simulink model "Copter_Plane_h2g_V10g"  (R2020b)
settings: Solver=ode1  StartTime=0.0  StopTime=6  FixedStep=dt  MaxStep=Ts  RelTol=1e-3
values from neighbouring files (symbols this model uses):
  HD = 180/pi    (= 57.2957795131)    [mode_data.m]
  POSCONTROL_ACC_Z_D = 0.3    [data_devg2.m]
  POSCONTROL_ACC_Z_P = 0.9    [data_devg2.m]
  POSCONTROL_VEL_XY_D = 0.12    [data_devg2.m]
  POSCONTROL_VEL_XY_P = 1.1    [data_devg2.m]
undefined symbols (not defined in the file or in its folder): accel_target, attitude_target_euler_angle, center_WP, curr_pos, curr_vel, GRAVITY_MSS, gyro_x, gyro_y, gyro_z, J, k_aileron, k_aileronL, k_aileronR, k_elevator, k_flap, k_rudder, m_kg, Newton, pid_vel_xy_derivative, pid_vel_xy_input, pid_vel_xy_integrator, pitch, pos_target, pwm_out, pwm_tail, Raphson, rate_target_ang_vel, roll, tail_tilt, Vehicle, vel_desired, vel_target, yaw
libraries: sharedutil x11, sharedtransform x5, shared6dofsys x3, simulink x2, aerolibasang x1
(part 4 of 5)

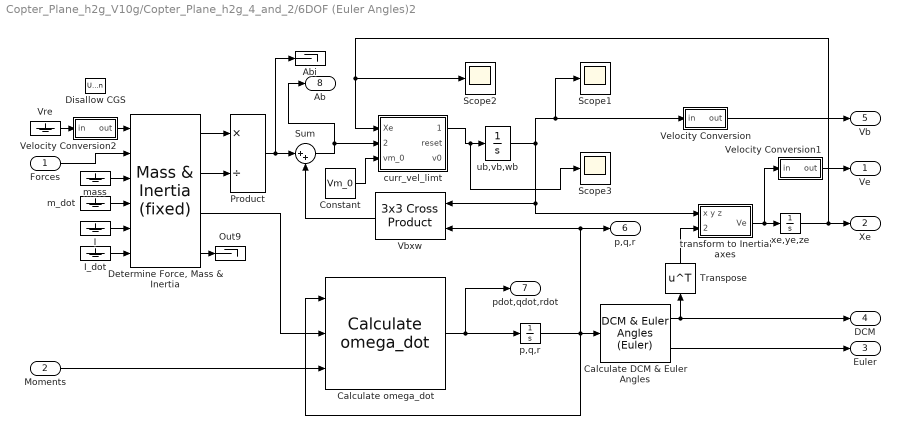
== system Copter_Plane_h2g_V10g/Copter_Plane_h2g_4_and_2/6DOF (Euler Angles)2 ==
  Forces : Inport  Unit=N  PortDimensions=3
  Moments : Inport  Port=2  Unit=N*m  PortDimensions=3
  Abi : Terminator
  Calculate DCM & Euler Angles : shared6dofsys/DCM & Euler Angles (Euler)  aMode=aMode
      settings: SourceProductBaseCode=AE,PW,MT,UV,VE,VP
  Calculate omega_dot : shared6dofsys/Calculate omega_dot  aMode=aMode
      settings: SourceProductBaseCode=AE,PW,MT,UV,VE,VP
  Constant : Constant  Value=Vm_0
  "Determine Force, Mass & Inertia" : shared6dofsys/Mass & Inertia (fixed)  aMode=aMode
      settings: SourceProductBaseCode=AE,PW,MT,UV,VE,VP
  Disallow CGS : UnitConfiguration  UnitSystemsStr=English,SI,SI (extended)  AllowAllUnitSystems=off
  I : Ground
  I_dot : Ground
  Out9 : Terminator
  Product : Product  Inputs=*/  SaturateOnIntegerOverflow=on  OutDataTypeStr=Inherit: Same as first input
  Scope1 : Scope
  Scope2 : Scope
  Scope3 : Scope
  Sum : Sum  Inputs=|++  SaturateOnIntegerOverflow=on
  Transpose : Math  Operator=transpose  SignedPower=on  SaturateOnIntegerOverflow=on
  Vbxw : sharedutil/3x3 Cross Product  aMode=aMode
      settings: SourceProductBaseCode=AE,PW,MT,UV,VE,VP
  Velocity Conversion : Subsystem
  Velocity Conversion1 : Subsystem
  Velocity Conversion2 : Subsystem
  Vre : Ground
  curr_vel_limt : MATLAB Function  TreatAsAtomicUnit=on
  m_dot : Ground
  mass : Ground
  "p,q,r " : Integrator  InitialCondition=pm_0  ContinuousStateAttributes=pm_statename
  "transform to Inertial axes " : Subsystem  mask(Vector Transformation){}
      mask Display: disp('L_EB')
  ub,vb,wb : Integrator  InitialCondition=Vm_0  UpperSaturationLimit=[inf inf 0]  ContinuousStateAttributes=Vm_statename
  xe,ye,ze : Integrator  InitialCondition=xme_0  ContinuousStateAttributes=xme_statename
  Ve : Outport  Unit=m/s  VectorParamsAs1DForOutWhenUnconnected=off
  Xe : Outport  Port=2  Unit=m  VectorParamsAs1DForOutWhenUnconnected=off
  Euler : Outport  Port=3  Unit=rad  VectorParamsAs1DForOutWhenUnconnected=off
  DCM : Outport  Port=4  Unit=1  VectorParamsAs1DForOutWhenUnconnected=off
  Vb : Outport  Port=5  Unit=m/s  VectorParamsAs1DForOutWhenUnconnected=off
  p,q,r : Outport  Port=6  Unit=rad/s  VectorParamsAs1DForOutWhenUnconnected=off
  pdot,qdot,rdot : Outport  Port=7  Unit=rad/s^2  VectorParamsAs1DForOutWhenUnconnected=off
  Ab : Outport  Port=8  Unit=m/s^2  VectorParamsAs1DForOutWhenUnconnected=off
  wires:
  Velocity Conversion1/1(out) -> Ve/1
  Sum/1 -> Ab/1, curr_vel_limt/2(accel_in)
  ub,vb,wb/1 -> "transform to Inertial axes "/1(x y z), Vbxw/1, Scope1/1, Velocity Conversion/1(in)
  Velocity Conversion/1(out) -> Vb/1
  Velocity Conversion2/1(out) -> "Determine Force, Mass & Inertia"/1
  Vre/1 -> Velocity Conversion2/1(in)
  "Determine Force, Mass & Inertia"/1 -> Product/1
  I_dot/1 -> "Determine Force, Mass & Inertia"/6
  I/1 -> "Determine Force, Mass & Inertia"/5
  Calculate omega_dot/1 -> "p,q,r "/1, pdot,qdot,rdot/1
  "Determine Force, Mass & Inertia"/4 -> Out9/1
  m_dot/1 -> "Determine Force, Mass & Inertia"/4
  "Determine Force, Mass & Inertia"/2 -> Product/2
  mass/1 -> "Determine Force, Mass & Inertia"/3
  Transpose/1 -> "transform to Inertial axes "/2(transform coefficients)
  Calculate DCM & Euler Angles/1 -> Transpose/1, DCM/1
  Product/1 -> Sum/1, Abi/1
  Forces/1 -> "Determine Force, Mass & Inertia"/2
  Moments/1 -> Calculate omega_dot/3
  "p,q,r "/1 -> Calculate DCM & Euler Angles/1, Calculate omega_dot/1, p,q,r/1, Vbxw/2
  "transform to Inertial axes "/1(Ve) -> xe,ye,ze/1, Velocity Conversion1/1(in)
  xe,ye,ze/1 -> Scope2/1, curr_vel_limt/1(Xe), Xe/1
  Vbxw/1 -> Sum/2
  Calculate DCM & Euler Angles/2 -> Euler/1
  "Determine Force, Mass & Inertia"/3 -> Calculate omega_dot/2
  curr_vel_limt/1(accel_o) -> Scope3/1, ub,vb,wb/1
  Constant/1 -> curr_vel_limt/3(vm_0)

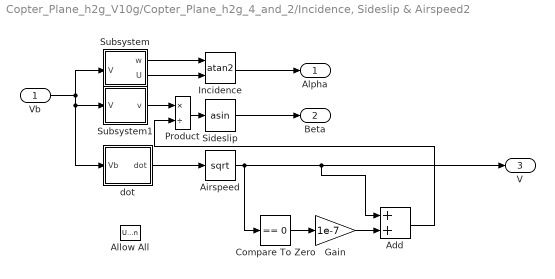
== system Copter_Plane_h2g_V10g/Copter_Plane_h2g_4_and_2/Incidence, Sideslip & Airspeed2 ==
  Vb : Inport
  Add : Sum
  Airspeed : Sqrt  AlgorithmType=Newton-Raphson  SaturateOnIntegerOverflow=on
  Allow All : UnitConfiguration  UnitSystemsStr=English,SI,SI (extended)  AllowAllUnitSystems=off
  Compare To Zero : simulink/Logic and Bit Operations/Compare To Zero  relop===  OutDataTypeStr=boolean
  Gain : Gain  Gain=1e-7
  Incidence : Trigonometry  Operator=atan2
  Product : Product  Inputs=*/  SaturateOnIntegerOverflow=on  OutDataTypeStr=Inherit: Same as first input
  Sideslip : Trigonometry  Operator=asin
  Subsystem : Subsystem
  Subsystem1 : Subsystem
  dot : Subsystem
  Alpha : Outport  Unit=rad  InitialOutput=0  VectorParamsAs1DForOutWhenUnconnected=off
  Beta : Outport  Port=2  Unit=rad  InitialOutput=0  VectorParamsAs1DForOutWhenUnconnected=off
  V : Outport  Port=3  InitialOutput=0  VectorParamsAs1DForOutWhenUnconnected=off
  wires:
  Product/1 -> Sideslip/1
  Subsystem/1(w) -> Incidence/1
  Subsystem/2(U) -> Incidence/2
  dot/1(dot) -> Airspeed/1
  Airspeed/1 -> Compare To Zero/1, Add/1, V/1
  Incidence/1 -> Alpha/1
  Vb/1 -> Subsystem/1(V), Subsystem1/1(V), dot/1(Vb)
  Sideslip/1 -> Beta/1
  Subsystem1/1(v) -> Product/1
  Compare To Zero/1 -> Gain/1
  Gain/1 -> Add/2
  Add/1 -> Product/2

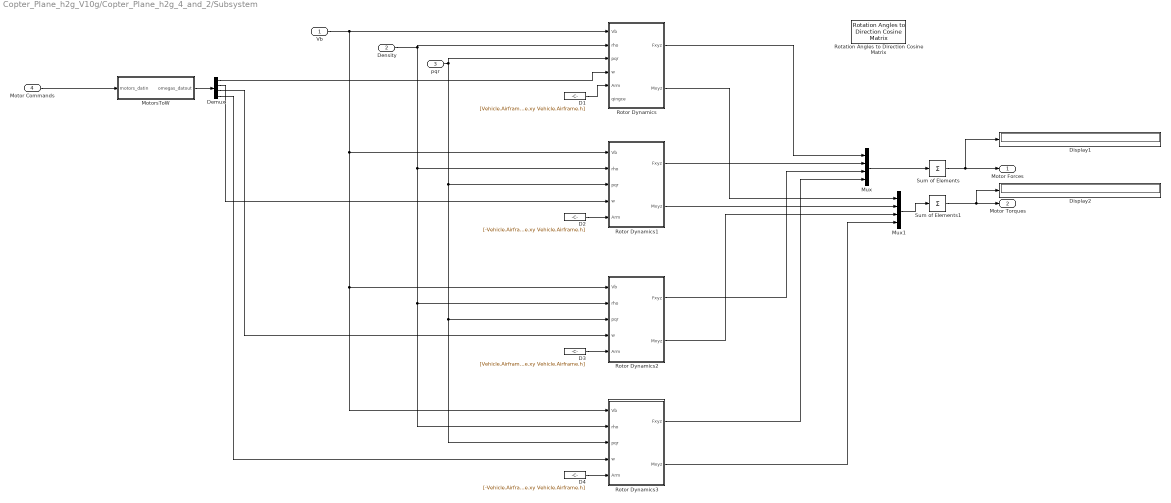
== system Copter_Plane_h2g_V10g/Copter_Plane_h2g_4_and_2/Subsystem ==
  Vb : Inport
  Density : Inport  Port=2
  pqr : Inport  Port=3
  Motor Commands : Inport  Port=4
  D1 : Constant  Value=[Vehicle.Airframe.xy +Vehicle.Airframe.xy Vehicle.Airframe.h]
  D2 : Constant  Value=[-Vehicle.Airframe.xy -Vehicle.Airframe.xy Vehicle.Airframe.h]
  D3 : Constant  Value=[Vehicle.Airframe.xy -Vehicle.Airframe.xy Vehicle.Airframe.h]
  D4 : Constant  Value=[-Vehicle.Airframe.xy Vehicle.Airframe.xy Vehicle.Airframe.h]
  Demux : Demux
  Display1 : Display
  Display2 : Display
  MotorsToW : Subsystem
  Mux : Mux
  Mux1 : Mux
  Rotation Angles to Direction Cosine Matrix : sharedtransform/Rotation Angles to Direction Cosine Matrix  rotationOrder=YZX  aMode=aMode
      settings: SourceProductBaseCode=AE,PW,MT,UV,VE,VP
  Rotor Dynamics : Subsystem  AncestorBlock=dynamicsLibrary/Rotor Dynamics  TreatAsAtomicUnit=on
      mask init:
      | aeroicon('aeroblk');
      settings: RTWFcnNameOpts=Use subsystem name  RTWFileNameOpts=Use function name
  Rotor Dynamics1 : Subsystem  AncestorBlock=dynamicsLibrary/Rotor Dynamics  TreatAsAtomicUnit=on
      mask init:
      | aeroicon('aeroblk');
      settings: RTWFcnNameOpts=Use subsystem name  RTWFileNameOpts=Use function name
  Rotor Dynamics2 : Subsystem  AncestorBlock=dynamicsLibrary/Rotor Dynamics  TreatAsAtomicUnit=on
      mask init:
      | aeroicon('aeroblk');
      settings: RTWFcnNameOpts=Use subsystem name  RTWFileNameOpts=Use function name
  Rotor Dynamics3 : Subsystem  AncestorBlock=dynamicsLibrary/Rotor Dynamics  TreatAsAtomicUnit=on
      mask init:
      | aeroicon('aeroblk');
      settings: RTWFcnNameOpts=Use subsystem name  RTWFileNameOpts=Use function name
  Sum of Elements : Sum  Inputs=+  CollapseMode=Specified dimension  CollapseDim=2
  Sum of Elements1 : Sum  Inputs=+  CollapseMode=Specified dimension  CollapseDim=2
  Motor Forces : Outport  Unit=N  VectorParamsAs1DForOutWhenUnconnected=off
  Motor Torques : Outport  Port=2  Unit=N*m  VectorParamsAs1DForOutWhenUnconnected=off
  wires:
  D4/1 -> Rotor Dynamics3/5(Arm)
  Sum of Elements1/1 -> Display2/1, Motor Torques/1
  D3/1 -> Rotor Dynamics2/5(Arm)
  Sum of Elements/1 -> Display1/1, Motor Forces/1
  D1/1 -> Rotor Dynamics/5(Arm)
  Mux1/1 -> Sum of Elements1/1
  Mux/1 -> Sum of Elements/1
  D2/1 -> Rotor Dynamics1/5(Arm)
  Motor Commands/1 -> MotorsToW/1(motors_datin)
  MotorsToW/1(omegas_datout) -> Demux/1
  Vb/1 -> Rotor Dynamics/1(Vb), Rotor Dynamics2/1(Vb), Rotor Dynamics3/1(Vb), Rotor Dynamics1/1(Vb)
  Density/1 -> Rotor Dynamics/2(rho), Rotor Dynamics2/2(rho), Rotor Dynamics3/2(rho), Rotor Dynamics1/2(rho)
  pqr/1 -> Rotor Dynamics/3(pqr), Rotor Dynamics2/3(pqr), Rotor Dynamics3/3(pqr), Rotor Dynamics1/3(pqr)
  Demux/1 -> Rotor Dynamics/4(w)
  Demux/2 -> Rotor Dynamics1/4(w)
  Demux/3 -> Rotor Dynamics2/4(w)
  Demux/4 -> Rotor Dynamics3/4(w)
  Rotor Dynamics/1(Fxyz) -> Mux/1
  Rotor Dynamics1/1(Fxyz) -> Mux/2
  Rotor Dynamics2/1(Fxyz) -> Mux/3
  Rotor Dynamics3/1(Fxyz) -> Mux/4
  Rotor Dynamics1/2(Mxyz) -> Mux1/2
  Rotor Dynamics2/2(Mxyz) -> Mux1/3
  Rotor Dynamics/2(Mxyz) -> Mux1/1
  Rotor Dynamics3/2(Mxyz) -> Mux1/4

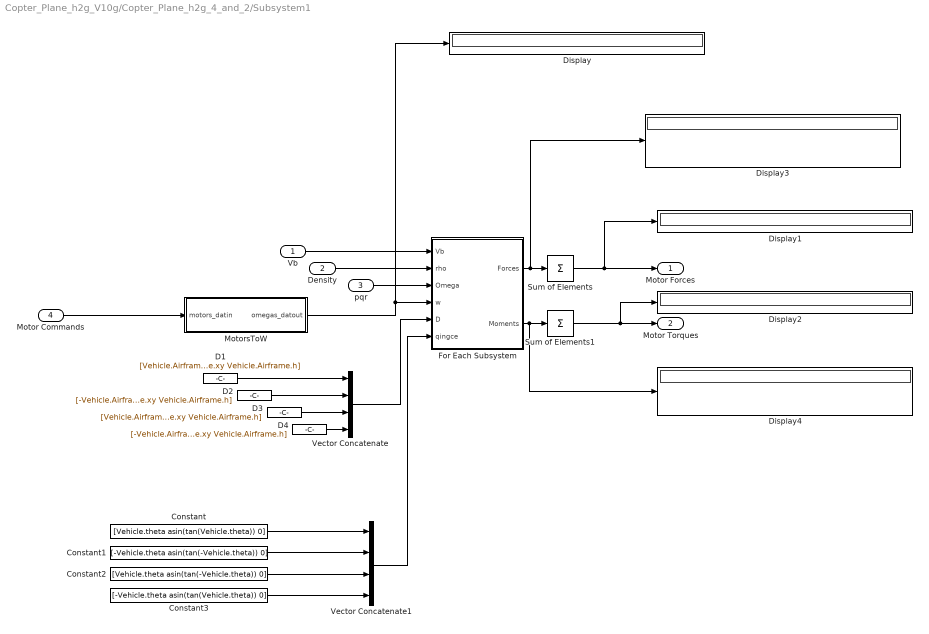
== system Copter_Plane_h2g_V10g/Copter_Plane_h2g_4_and_2/Subsystem1 ==
  Vb : Inport
  Density : Inport  Port=2
  pqr : Inport  Port=3
  Motor Commands : Inport  Port=4
  Constant : Constant  Value=[Vehicle.theta asin(tan(Vehicle.theta)) 0]
  Constant1 : Constant  Value=[-Vehicle.theta asin(tan(-Vehicle.theta)) 0]
  Constant2 : Constant  Value=[Vehicle.theta asin(tan(-Vehicle.theta)) 0]
  Constant3 : Constant  Value=[-Vehicle.theta asin(tan(Vehicle.theta)) 0]
  D1 : Constant  Value=[Vehicle.Airframe.xy +Vehicle.Airframe.xy Vehicle.Airframe.h]
  D2 : Constant  Value=[-Vehicle.Airframe.xy -Vehicle.Airframe.xy Vehicle.Airframe.h]
  D3 : Constant  Value=[Vehicle.Airframe.xy -Vehicle.Airframe.xy Vehicle.Airframe.h]
  D4 : Constant  Value=[-Vehicle.Airframe.xy Vehicle.Airframe.xy Vehicle.Airframe.h]
  Display{,1..4} (5 alike) : Display
  For Each Subsystem : Subsystem  TreatAsAtomicUnit=on
  MotorsToW : Subsystem
  Sum of Elements : Sum  Inputs=+  CollapseMode=Specified dimension  CollapseDim=2
  Sum of Elements1 : Sum  Inputs=+  CollapseMode=Specified dimension  CollapseDim=2
  Vector Concatenate : Concatenate  NumInputs=4  Mode=Multidimensional array  ConcatenateDimension=2
  Vector Concatenate1 : Concatenate  NumInputs=4  Mode=Multidimensional array  ConcatenateDimension=2
  Motor Forces : Outport  Unit=N  VectorParamsAs1DForOutWhenUnconnected=off
  Motor Torques : Outport  Port=2  Unit=N*m  VectorParamsAs1DForOutWhenUnconnected=off
  wires:
  Vector Concatenate/1 -> For Each Subsystem/5(D)
  Density/1 -> For Each Subsystem/2(rho)
  D4/1 -> Vector Concatenate/4
  Vb/1 -> For Each Subsystem/1(Vb)
  Sum of Elements1/1 -> Display2/1, Motor Torques/1
  D3/1 -> Vector Concatenate/3
  Sum of Elements/1 -> Display1/1, Motor Forces/1
  pqr/1 -> For Each Subsystem/3(Omega)
  D1/1 -> Vector Concatenate/1
  For Each Subsystem/2(Moments) -> Display4/1, Sum of Elements1/1
  For Each Subsystem/1(Forces) -> Display3/1, Sum of Elements/1
  D2/1 -> Vector Concatenate/2
  MotorsToW/1(omegas_datout) -> Display/1, For Each Subsystem/4(w)
  Motor Commands/1 -> MotorsToW/1(motors_datin)
  Vector Concatenate1/1 -> For Each Subsystem/6(qingce)
  Constant/1 -> Vector Concatenate1/1
  Constant1/1 -> Vector Concatenate1/2
  Constant2/1 -> Vector Concatenate1/3
  Constant3/1 -> Vector Concatenate1/4

== system Copter_Plane_h2g_V10g/Copter_Plane_h2g_4_and_2/6DOF (Euler Angles)2/Velocity Conversion ==
  in : Inport  Unit=m/s
  Unit Conversion : UnitConversion
  out : Outport  VectorParamsAs1DForOutWhenUnconnected=off
  wires:
  Unit Conversion/1 -> out/1
  in/1 -> Unit Conversion/1

== system Copter_Plane_h2g_V10g/Copter_Plane_h2g_4_and_2/6DOF (Euler Angles)2/Velocity Conversion1 ==
  in : Inport  Unit=m/s
  Unit Conversion : UnitConversion
  out : Outport  VectorParamsAs1DForOutWhenUnconnected=off
  wires:
  Unit Conversion/1 -> out/1
  in/1 -> Unit Conversion/1

== system Copter_Plane_h2g_V10g/Copter_Plane_h2g_4_and_2/6DOF (Euler Angles)2/Velocity Conversion2 ==
  in : Inport  Unit=m/s
  Unit Conversion : UnitConversion
  out : Outport  Unit=m/s  VectorParamsAs1DForOutWhenUnconnected=off
  wires:
  Unit Conversion/1 -> out/1
  in/1 -> Unit Conversion/1

== system Copter_Plane_h2g_V10g/Copter_Plane_h2g_4_and_2/6DOF (Euler Angles)2/transform to Inertial axes  ==
  x y z : Inport
  transform coefficients : Inport  Port=2
  Product : Product  Multiplication=Matrix(*)  InputSameDT=on  SaturateOnIntegerOverflow=on  OutDataTypeStr=Inherit: Same as first input
  Reshape1 : Reshape  OutputDimensionality=Column vector (2-D)
  Reshape2 : Reshape
  Ve : Outport  VectorParamsAs1DForOutWhenUnconnected=off
  wires:
  Reshape2/1 -> Ve/1
  Reshape1/1 -> Product/2
  x y z/1 -> Reshape1/1
  transform coefficients/1 -> Product/1
  Product/1 -> Reshape2/1

== system Copter_Plane_h2g_V10g/Copter_Plane_h2g_4_and_2/Incidence, Sideslip & Airspeed2/Subsystem ==
  V : Inport
  Demux1 : Demux  Outputs=3
      settings: DisplayOption=none
  Terminator : Terminator
  w : Outport  VectorParamsAs1DForOutWhenUnconnected=off
  U : Outport  Port=2  VectorParamsAs1DForOutWhenUnconnected=off
  wires:
  Demux1/3 -> w/1
  Demux1/2 -> Terminator/1
  V/1 -> Demux1/1
  Demux1/1 -> U/1

== system Copter_Plane_h2g_V10g/Copter_Plane_h2g_4_and_2/Incidence, Sideslip & Airspeed2/Subsystem1 ==
  V : Inport
  Demux1 : Demux  Outputs=3
      settings: DisplayOption=none
  Terminator : Terminator
  Terminator1 : Terminator
  v : Outport  VectorParamsAs1DForOutWhenUnconnected=off
  wires:
  Demux1/1 -> Terminator/1
  Demux1/3 -> Terminator1/1
  V/1 -> Demux1/1
  Demux1/2 -> v/1

== system Copter_Plane_h2g_V10g/Copter_Plane_h2g_4_and_2/Incidence, Sideslip & Airspeed2/dot ==
  Vb : Inport
  Demux1 : Demux  Outputs=3
  Product : Product  RndMeth=Zero
  Product1 : Product  RndMeth=Zero
  Product2 : Product  RndMeth=Zero
  Sum : Sum  Inputs=+++
  dot : Outport  VectorParamsAs1DForOutWhenUnconnected=off
  wires:
  Product2/1 -> Sum/3
  Demux1/3 -> Product2/2, Product2/1
  Product/1 -> Sum/1
  Product1/1 -> Sum/2
  Sum/1 -> dot/1
  Vb/1 -> Demux1/1
  Demux1/1 -> Product/2, Product/1
  Demux1/2 -> Product1/1, Product1/2

== system Copter_Plane_h2g_V10g/Copter_Plane_h2g_4_and_2/Subsystem/MotorsToW ==
  motors_datin : Inport
  Motordirections1 : Gain  Gain=[1 1 -1 -1]  ParamDataTypeStr=single  OutDataTypeStr=Inherit: Inherit via back propagation  SaturateOnIntegerOverflow=on
  Saturation5 : Saturate  UpperLimit=1  LowerLimit=realmin  OutDataTypeStr=Inherit: Inherit via back propagation
  motorsToW2_Gain : Gain  Gain=Vehicle.Motor.commandToWGain  ParamDataTypeStr=single  OutDataTypeStr=Inherit: Inherit via back propagation  SaturateOnIntegerOverflow=on
  motorsToW2_Gain1 : Gain  Gain=2*pi/60  ParamDataTypeStr=single  OutDataTypeStr=Inherit: Inherit via back propagation  SaturateOnIntegerOverflow=on
  omegas_datout : Outport  VectorParamsAs1DForOutWhenUnconnected=off
  wires:
  Saturation5/1 -> Motordirections1/1
  Motordirections1/1 -> motorsToW2_Gain/1
  motors_datin/1 -> Saturation5/1
  motorsToW2_Gain/1 -> motorsToW2_Gain1/1
  motorsToW2_Gain1/1 -> omegas_datout/1

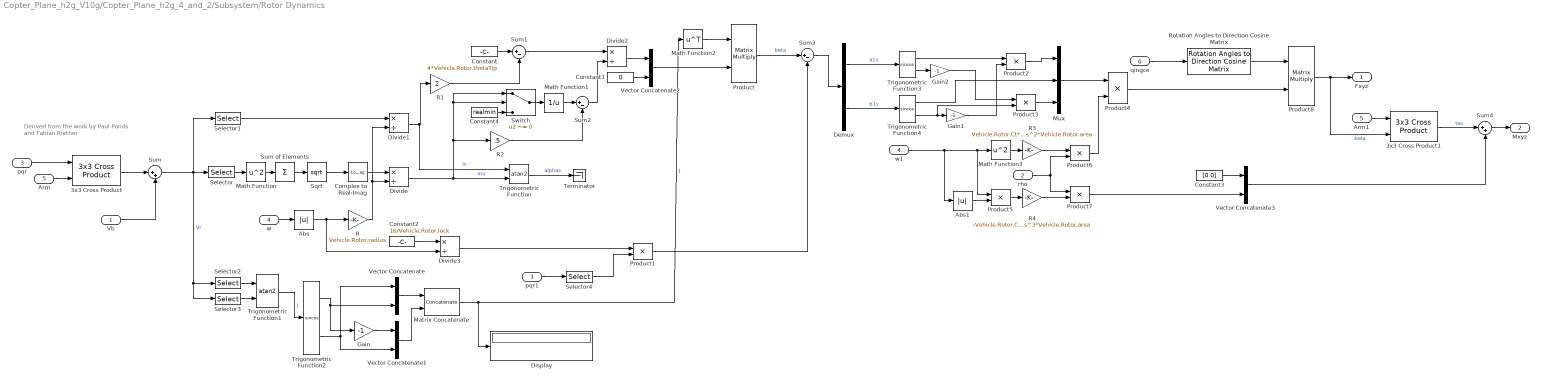
== system Copter_Plane_h2g_V10g/Copter_Plane_h2g_4_and_2/Subsystem/Rotor Dynamics ==
  note: Derived from the work by Paul Ponds
      | and Fabian Riether
  Vb : Inport  PortDimensions=3
  rho : Inport  Port=2  PortDimensions=1
  pqr : Inport  Port=3  PortDimensions=3
  w : Inport  Port=4  PortDimensions=[1 1]
  Arm : Inport  Port=5  PortDimensions=[3 1]
  qingce : Inport  Port=6  PortDimensions=[3 1]
  3x3 Cross Product : sharedutil/3x3 Cross Product  aMode=aMode
      settings: SourceProductBaseCode=AE,PW,MT,UV,VE,VP
  3x3 Cross Product1 : sharedutil/3x3 Cross Product  aMode=aMode
      settings: SourceProductBaseCode=AE,PW,MT,UV,VE,VP
  Abs : Abs
  Abs1 : Abs
  Arm1 : InportShadow  Port=5  PortDimensions=[3 1]
  Complex to Real-Imag : ComplexToRealImag  Output=Real
  Constant : Constant  Value=4*Vehicle.Rotor.thetaTip
  Constant1 : Constant  Value=0
  Constant2 : Constant  Value=16/Vehicle.Rotor.lock
  Constant3 : Constant  Value=[0 0]
  Constant4 : Constant  Value=realmin
  Demux : Demux  Outputs=2
  Display : Display
  Divide{,1..3} (4 alike) : Product  Inputs=*/
  Gain : Gain  Gain=-1
  Gain1 : Gain  Gain=-1
  Gain2 : Gain  Gain=-1
  Math Function : Math  Operator=square  SignedPower=on  SaturateOnIntegerOverflow=on
  Math Function1 : Math  Operator=reciprocal  SignedPower=on  SaturateOnIntegerOverflow=on
  Math Function2 : Math  Operator=transpose  SignedPower=on  SaturateOnIntegerOverflow=on
  Math Function3 : Math  Operator=square  SignedPower=on  SaturateOnIntegerOverflow=on
  Matrix Concatenate : Concatenate  Mode=Multidimensional array  ConcatenateDimension=2
  Mux : Mux  Inputs=3
  Product : Product  Multiplication=Matrix(*)
  Product{1..7} (7 alike) : Product
  Product8 : Product  Multiplication=Matrix(*)
  R : Gain  Gain=Vehicle.Rotor.radius
  R1 : Gain  Gain=2
  R2 : Gain  Gain=.5
  R3 : Gain  Gain=Vehicle.Rotor.Ct*Vehicle.Rotor.radius^2*Vehicle.Rotor.area
  R4 : Gain  Gain=-Vehicle.Rotor.Cq*Vehicle.Rotor.radius^3*Vehicle.Rotor.area
  Rotation Angles to Direction Cosine Matrix : sharedtransform/Rotation Angles to Direction Cosine Matrix  rotationOrder=YXZ  aMode=aMode
      settings: SourceProductBaseCode=AE,PW,MT,UV,VE,VP
  Selector : Selector  InputPortWidth=3  IndexOptions=Index vector (dialog)  Indices=[1 2]  OutputSizes=1
  Selector1 : Selector  InputPortWidth=3  IndexOptions=Index vector (dialog)  Indices=[3]  OutputSizes=1
  Selector2 : Selector  InputPortWidth=3  IndexOptions=Index vector (dialog)  Indices=[2]  OutputSizes=1
  Selector3 : Selector  InputPortWidth=3  IndexOptions=Index vector (dialog)  Indices=[1]  OutputSizes=1
  Selector4 : Selector  InputPortWidth=3  IndexOptions=Index vector (dialog)  Indices=[2 1]  OutputSizes=1
  Sqrt : Sqrt  OutputSignalType=complex  SaturateOnIntegerOverflow=on
  Sum : Sum  Inputs=|++
  Sum of Elements : Sum  Inputs=+
  Sum1 : Sum  Inputs=|+-
  Sum2 : Sum  Inputs=|+-
  Sum3 : Sum  Inputs=|+-
  Sum4 : Sum  Inputs=|++
  Switch : Switch  Criteria=u2 ~= 0
  Terminator : Terminator
  Trigonometric Function : Trigonometry  Operator=atan2
  Trigonometric Function1 : Trigonometry  Operator=atan2
  Trigonometric Function2 : Trigonometry  Operator=sincos
  Trigonometric Function3 : Trigonometry  Operator=sincos
  Trigonometric Function4 : Trigonometry  Operator=sincos
  Vector Concatenate{,1..3} (4 alike) : Concatenate
  pqr1 : InportShadow  Port=3  PortDimensions=3
  w1 : InportShadow  Port=4  PortDimensions=[1 1]
  Fxyz : Outport  PortDimensions=[3 1]  VectorParamsAs1DForOutWhenUnconnected=off
  Mxyz : Outport  Port=2  PortDimensions=[3 1]  VectorParamsAs1DForOutWhenUnconnected=off
  wires:
  Complex to Real-Imag/1 -> Divide/1
  Sqrt/1 -> Complex to Real-Imag/1
  Constant4/1 -> Switch/3
  Switch/1 -> Math Function1/1
  Product1/1 -> Sum3/2
  rho/1 -> Product7/1, Product6/2
  Product7/1 -> Vector Concatenate3/2
  Product6/1 -> Product4/2
  Sum4/1 -> Mxyz/1
  3x3 Cross Product1/1 -> Sum4/1  "tau"
  Product4/1 -> Product8/2
  Arm1/1 -> 3x3 Cross Product1/1
  Vector Concatenate3/1 -> Sum4/2
  Constant3/1 -> Vector Concatenate3/1
  R4/1 -> Product7/2
  Product5/1 -> R4/1
  Abs1/1 -> Product5/2
  R3/1 -> Product6/1
  Mux/1 -> Product4/1
  Gain2/1 -> Product3/1
  Product3/1 -> Mux/3
  Trigonometric Function3/2 -> Gain2/1
  Trigonometric Function4/1 -> Mux/2
  Product2/1 -> Mux/1
  Trigonometric Function3/1 -> Product2/1
  Gain1/1 -> Product2/2
  Trigonometric Function4/2 -> Gain1/1, Product3/2
  Demux/2 -> Trigonometric Function4/1  "b1s"
  Demux/1 -> Trigonometric Function3/1  "a1s"
  Sum3/1 -> Demux/1
  Math Function3/1 -> R3/1
  w1/1 -> Math Function3/1, Product5/1, Abs1/1
  Divide3/1 -> Product1/1
  Abs/1 -> R/1, Divide3/2
  Selector4/1 -> Product1/2
  pqr1/1 -> Selector4/1
  Constant2/1 -> Divide3/1
  Product/1 -> Sum3/1  "beta"
  Math Function2/1 -> Product/1
  Vector Concatenate2/1 -> Product/2
  Constant1/1 -> Vector Concatenate2/2
  Divide2/1 -> Vector Concatenate2/1
  Sum2/1 -> Divide2/2
  R2/1 -> Sum2/2
  Math Function1/1 -> Sum2/1
  Sum1/1 -> Divide2/1
  R1/1 -> Sum1/2
  Constant/1 -> Sum1/1
  Matrix Concatenate/1 -> Display/1, Math Function2/1  "J"
  Vector Concatenate1/1 -> Matrix Concatenate/2
  Vector Concatenate/1 -> Matrix Concatenate/1
  Trigonometric Function2/1 -> Gain/1, Vector Concatenate/2
  Gain/1 -> Vector Concatenate1/1
  Trigonometric Function2/2 -> Vector Concatenate/1, Vector Concatenate1/2
  Trigonometric Function1/1 -> Trigonometric Function2/1  "j"
  Selector3/1 -> Trigonometric Function1/2
  Selector2/1 -> Trigonometric Function1/1
  Trigonometric Function/1 -> Terminator/1  "alphas"
  Divide1/1 -> Trigonometric Function/1, R1/1  "lc"
  Selector1/1 -> Divide1/1
  Divide/1 -> Trigonometric Function/2, Switch/1, Switch/2, R2/1  "mu"
  R/1 -> Divide/2, Divide1/2
  w/1 -> Abs/1
  Arm/1 -> 3x3 Cross Product/2
  pqr/1 -> 3x3 Cross Product/1
  Sum of Elements/1 -> Sqrt/1
  Math Function/1 -> Sum of Elements/1
  Selector/1 -> Math Function/1
  Sum/1 -> Selector/1, Selector1/1, Selector2/1, Selector3/1  "Vr"
  Vb/1 -> Sum/2
  3x3 Cross Product/1 -> Sum/1
  Rotation Angles to Direction Cosine Matrix/1 -> Product8/1
  Product8/1 -> 3x3 Cross Product1/2, Fxyz/1  "beta"
  qingce/1 -> Rotation Angles to Direction Cosine Matrix/1

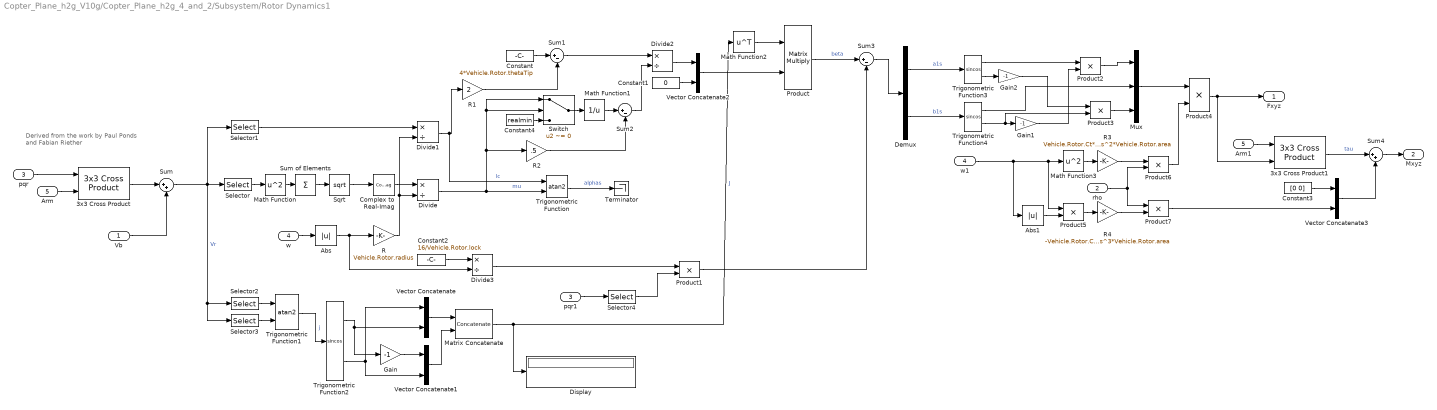
== system Copter_Plane_h2g_V10g/Copter_Plane_h2g_4_and_2/Subsystem/Rotor Dynamics1 ==
  note: Derived from the work by Paul Ponds
      | and Fabian Riether
  Vb : Inport  PortDimensions=3
  rho : Inport  Port=2  PortDimensions=1
  pqr : Inport  Port=3  PortDimensions=3
  w : Inport  Port=4  PortDimensions=[1 1]
  Arm : Inport  Port=5  PortDimensions=[3 1]
  3x3 Cross Product : sharedutil/3x3 Cross Product  aMode=aMode
      settings: SourceProductBaseCode=AE,PW,MT,UV,VE,VP
  3x3 Cross Product1 : sharedutil/3x3 Cross Product  aMode=aMode
      settings: SourceProductBaseCode=AE,PW,MT,UV,VE,VP
  Abs : Abs
  Abs1 : Abs
  Arm1 : InportShadow  Port=5  PortDimensions=[3 1]
  Complex to Real-Imag : ComplexToRealImag  Output=Real
  Constant : Constant  Value=4*Vehicle.Rotor.thetaTip
  Constant1 : Constant  Value=0
  Constant2 : Constant  Value=16/Vehicle.Rotor.lock
  Constant3 : Constant  Value=[0 0]
  Constant4 : Constant  Value=realmin
  Demux : Demux  Outputs=2
  Display : Display
  Divide{,1..3} (4 alike) : Product  Inputs=*/
  Gain : Gain  Gain=-1
  Gain1 : Gain  Gain=-1
  Gain2 : Gain  Gain=-1
  Math Function : Math  Operator=square  SignedPower=on  SaturateOnIntegerOverflow=on
  Math Function1 : Math  Operator=reciprocal  SignedPower=on  SaturateOnIntegerOverflow=on
  Math Function2 : Math  Operator=transpose  SignedPower=on  SaturateOnIntegerOverflow=on
  Math Function3 : Math  Operator=square  SignedPower=on  SaturateOnIntegerOverflow=on
  Matrix Concatenate : Concatenate  Mode=Multidimensional array  ConcatenateDimension=2
  Mux : Mux  Inputs=3
  Product : Product  Multiplication=Matrix(*)
  Product{1..7} (7 alike) : Product
  R : Gain  Gain=Vehicle.Rotor.radius
  R1 : Gain  Gain=2
  R2 : Gain  Gain=.5
  R3 : Gain  Gain=Vehicle.Rotor.Ct*Vehicle.Rotor.radius^2*Vehicle.Rotor.area
  R4 : Gain  Gain=-Vehicle.Rotor.Cq*Vehicle.Rotor.radius^3*Vehicle.Rotor.area
  Selector : Selector  InputPortWidth=3  IndexOptions=Index vector (dialog)  Indices=[1 2]  OutputSizes=1
  Selector1 : Selector  InputPortWidth=3  IndexOptions=Index vector (dialog)  Indices=[3]  OutputSizes=1
  Selector2 : Selector  InputPortWidth=3  IndexOptions=Index vector (dialog)  Indices=[2]  OutputSizes=1
  Selector3 : Selector  InputPortWidth=3  IndexOptions=Index vector (dialog)  Indices=[1]  OutputSizes=1
  Selector4 : Selector  InputPortWidth=3  IndexOptions=Index vector (dialog)  Indices=[2 1]  OutputSizes=1
  Sqrt : Sqrt  OutputSignalType=complex  SaturateOnIntegerOverflow=on
  Sum : Sum  Inputs=|++
  Sum of Elements : Sum  Inputs=+
  Sum1 : Sum  Inputs=|+-
  Sum2 : Sum  Inputs=|+-
  Sum3 : Sum  Inputs=|+-
  Sum4 : Sum  Inputs=|++
  Switch : Switch  Criteria=u2 ~= 0
  Terminator : Terminator
  Trigonometric Function : Trigonometry  Operator=atan2
  Trigonometric Function1 : Trigonometry  Operator=atan2
  Trigonometric Function2 : Trigonometry  Operator=sincos
  Trigonometric Function3 : Trigonometry  Operator=sincos
  Trigonometric Function4 : Trigonometry  Operator=sincos
  Vector Concatenate{,1..3} (4 alike) : Concatenate
  pqr1 : InportShadow  Port=3  PortDimensions=3
  w1 : InportShadow  Port=4  PortDimensions=[1 1]
  Fxyz : Outport  PortDimensions=[3 1]  VectorParamsAs1DForOutWhenUnconnected=off
  Mxyz : Outport  Port=2  PortDimensions=[3 1]  VectorParamsAs1DForOutWhenUnconnected=off
  wires:
  3x3 Cross Product/1 -> Sum/1
  Vb/1 -> Sum/2
  Sum/1 -> Selector3/1, Selector2/1, Selector1/1, Selector/1  "Vr"
  Selector/1 -> Math Function/1
  Math Function/1 -> Sum of Elements/1
  Sum of Elements/1 -> Sqrt/1
  pqr/1 -> 3x3 Cross Product/1
  Arm/1 -> 3x3 Cross Product/2
  w/1 -> Abs/1
  R/1 -> Divide1/2, Divide/2
  Divide/1 -> R2/1, Switch/2, Switch/1, Trigonometric Function/2  "mu"
  Selector1/1 -> Divide1/1
  Divide1/1 -> R1/1, Trigonometric Function/1  "lc"
  Trigonometric Function/1 -> Terminator/1  "alphas"
  Selector2/1 -> Trigonometric Function1/1
  Selector3/1 -> Trigonometric Function1/2
  Trigonometric Function1/1 -> Trigonometric Function2/1  "j"
  Trigonometric Function2/2 -> Vector Concatenate1/2, Vector Concatenate/1
  Gain/1 -> Vector Concatenate1/1
  Trigonometric Function2/1 -> Vector Concatenate/2, Gain/1
  Vector Concatenate/1 -> Matrix Concatenate/1
  Vector Concatenate1/1 -> Matrix Concatenate/2
  Matrix Concatenate/1 -> Math Function2/1, Display/1  "J"
  Constant/1 -> Sum1/1
  R1/1 -> Sum1/2
  Sum1/1 -> Divide2/1
  Math Function1/1 -> Sum2/1
  R2/1 -> Sum2/2
  Sum2/1 -> Divide2/2
  Divide2/1 -> Vector Concatenate2/1
  Constant1/1 -> Vector Concatenate2/2
  Vector Concatenate2/1 -> Product/2
  Math Function2/1 -> Product/1
  Product/1 -> Sum3/1  "beta"
  Constant2/1 -> Divide3/1
  pqr1/1 -> Selector4/1
  Selector4/1 -> Product1/2
  Abs/1 -> Divide3/2, R/1
  Divide3/1 -> Product1/1
  w1/1 -> Abs1/1, Product5/1, Math Function3/1
  Math Function3/1 -> R3/1
  Sum3/1 -> Demux/1
  Demux/1 -> Trigonometric Function3/1  "a1s"
  Demux/2 -> Trigonometric Function4/1  "b1s"
  Trigonometric Function4/2 -> Product3/2, Gain1/1
  Gain1/1 -> Product2/2
  Trigonometric Function3/1 -> Product2/1
  Product2/1 -> Mux/1
  Trigonometric Function4/1 -> Mux/2
  Trigonometric Function3/2 -> Gain2/1
  Product3/1 -> Mux/3
  Gain2/1 -> Product3/1
  Mux/1 -> Product4/1
  R3/1 -> Product6/1
  Abs1/1 -> Product5/2
  Product5/1 -> R4/1
  R4/1 -> Product7/2
  Constant3/1 -> Vector Concatenate3/1
  Vector Concatenate3/1 -> Sum4/2
  Arm1/1 -> 3x3 Cross Product1/1
  Product4/1 -> 3x3 Cross Product1/2, Fxyz/1
  3x3 Cross Product1/1 -> Sum4/1  "tau"
  Sum4/1 -> Mxyz/1
  Product6/1 -> Product4/2
  Product7/1 -> Vector Concatenate3/2
  rho/1 -> Product6/2, Product7/1
  Product1/1 -> Sum3/2
  Switch/1 -> Math Function1/1
  Constant4/1 -> Switch/3
  Sqrt/1 -> Complex to Real-Imag/1
  Complex to Real-Imag/1 -> Divide/1

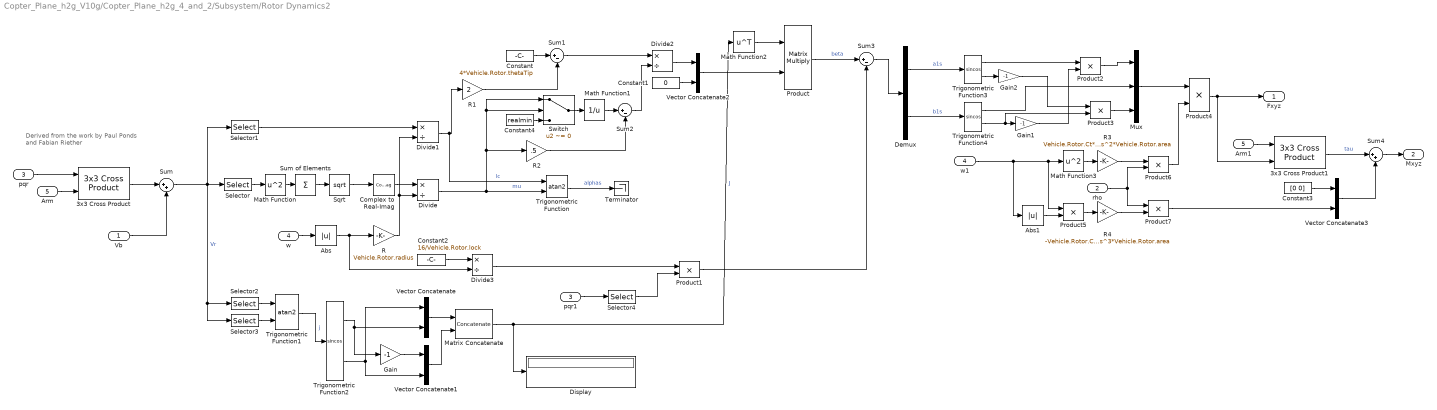
== system Copter_Plane_h2g_V10g/Copter_Plane_h2g_4_and_2/Subsystem/Rotor Dynamics2 ==
  note: Derived from the work by Paul Ponds
      | and Fabian Riether
  Vb : Inport  PortDimensions=3
  rho : Inport  Port=2  PortDimensions=1
  pqr : Inport  Port=3  PortDimensions=3
  w : Inport  Port=4  PortDimensions=[1 1]
  Arm : Inport  Port=5  PortDimensions=[3 1]
  3x3 Cross Product : sharedutil/3x3 Cross Product  aMode=aMode
      settings: SourceProductBaseCode=AE,PW,MT,UV,VE,VP
  3x3 Cross Product1 : sharedutil/3x3 Cross Product  aMode=aMode
      settings: SourceProductBaseCode=AE,PW,MT,UV,VE,VP
  Abs : Abs
  Abs1 : Abs
  Arm1 : InportShadow  Port=5  PortDimensions=[3 1]
  Complex to Real-Imag : ComplexToRealImag  Output=Real
  Constant : Constant  Value=4*Vehicle.Rotor.thetaTip
  Constant1 : Constant  Value=0
  Constant2 : Constant  Value=16/Vehicle.Rotor.lock
  Constant3 : Constant  Value=[0 0]
  Constant4 : Constant  Value=realmin
  Demux : Demux  Outputs=2
  Display : Display
  Divide{,1..3} (4 alike) : Product  Inputs=*/
  Gain : Gain  Gain=-1
  Gain1 : Gain  Gain=-1
  Gain2 : Gain  Gain=-1
  Math Function : Math  Operator=square  SignedPower=on  SaturateOnIntegerOverflow=on
  Math Function1 : Math  Operator=reciprocal  SignedPower=on  SaturateOnIntegerOverflow=on
  Math Function2 : Math  Operator=transpose  SignedPower=on  SaturateOnIntegerOverflow=on
  Math Function3 : Math  Operator=square  SignedPower=on  SaturateOnIntegerOverflow=on
  Matrix Concatenate : Concatenate  Mode=Multidimensional array  ConcatenateDimension=2
  Mux : Mux  Inputs=3
  Product : Product  Multiplication=Matrix(*)
  Product{1..7} (7 alike) : Product
  R : Gain  Gain=Vehicle.Rotor.radius
  R1 : Gain  Gain=2
  R2 : Gain  Gain=.5
  R3 : Gain  Gain=Vehicle.Rotor.Ct*Vehicle.Rotor.radius^2*Vehicle.Rotor.area
  R4 : Gain  Gain=-Vehicle.Rotor.Cq*Vehicle.Rotor.radius^3*Vehicle.Rotor.area
  Selector : Selector  InputPortWidth=3  IndexOptions=Index vector (dialog)  Indices=[1 2]  OutputSizes=1
  Selector1 : Selector  InputPortWidth=3  IndexOptions=Index vector (dialog)  Indices=[3]  OutputSizes=1
  Selector2 : Selector  InputPortWidth=3  IndexOptions=Index vector (dialog)  Indices=[2]  OutputSizes=1
  Selector3 : Selector  InputPortWidth=3  IndexOptions=Index vector (dialog)  Indices=[1]  OutputSizes=1
  Selector4 : Selector  InputPortWidth=3  IndexOptions=Index vector (dialog)  Indices=[2 1]  OutputSizes=1
  Sqrt : Sqrt  OutputSignalType=complex  SaturateOnIntegerOverflow=on
  Sum : Sum  Inputs=|++
  Sum of Elements : Sum  Inputs=+
  Sum1 : Sum  Inputs=|+-
  Sum2 : Sum  Inputs=|+-
  Sum3 : Sum  Inputs=|+-
  Sum4 : Sum  Inputs=|++
  Switch : Switch  Criteria=u2 ~= 0
  Terminator : Terminator
  Trigonometric Function : Trigonometry  Operator=atan2
  Trigonometric Function1 : Trigonometry  Operator=atan2
  Trigonometric Function2 : Trigonometry  Operator=sincos
  Trigonometric Function3 : Trigonometry  Operator=sincos
  Trigonometric Function4 : Trigonometry  Operator=sincos
  Vector Concatenate{,1..3} (4 alike) : Concatenate
  pqr1 : InportShadow  Port=3  PortDimensions=3
  w1 : InportShadow  Port=4  PortDimensions=[1 1]
  Fxyz : Outport  PortDimensions=[3 1]  VectorParamsAs1DForOutWhenUnconnected=off
  Mxyz : Outport  Port=2  PortDimensions=[3 1]  VectorParamsAs1DForOutWhenUnconnected=off
  wires:
  Complex to Real-Imag/1 -> Divide/1
  Sqrt/1 -> Complex to Real-Imag/1
  Constant4/1 -> Switch/3
  Switch/1 -> Math Function1/1
  Product1/1 -> Sum3/2
  rho/1 -> Product7/1, Product6/2
  Product7/1 -> Vector Concatenate3/2
  Product6/1 -> Product4/2
  Sum4/1 -> Mxyz/1
  3x3 Cross Product1/1 -> Sum4/1  "tau"
  Product4/1 -> Fxyz/1, 3x3 Cross Product1/2
  Arm1/1 -> 3x3 Cross Product1/1
  Vector Concatenate3/1 -> Sum4/2
  Constant3/1 -> Vector Concatenate3/1
  R4/1 -> Product7/2
  Product5/1 -> R4/1
  Abs1/1 -> Product5/2
  R3/1 -> Product6/1
  Mux/1 -> Product4/1
  Gain2/1 -> Product3/1
  Product3/1 -> Mux/3
  Trigonometric Function3/2 -> Gain2/1
  Trigonometric Function4/1 -> Mux/2
  Product2/1 -> Mux/1
  Trigonometric Function3/1 -> Product2/1
  Gain1/1 -> Product2/2
  Trigonometric Function4/2 -> Gain1/1, Product3/2
  Demux/2 -> Trigonometric Function4/1  "b1s"
  Demux/1 -> Trigonometric Function3/1  "a1s"
  Sum3/1 -> Demux/1
  Math Function3/1 -> R3/1
  w1/1 -> Math Function3/1, Product5/1, Abs1/1
  Divide3/1 -> Product1/1
  Abs/1 -> R/1, Divide3/2
  Selector4/1 -> Product1/2
  pqr1/1 -> Selector4/1
  Constant2/1 -> Divide3/1
  Product/1 -> Sum3/1  "beta"
  Math Function2/1 -> Product/1
  Vector Concatenate2/1 -> Product/2
  Constant1/1 -> Vector Concatenate2/2
  Divide2/1 -> Vector Concatenate2/1
  Sum2/1 -> Divide2/2
  R2/1 -> Sum2/2
  Math Function1/1 -> Sum2/1
  Sum1/1 -> Divide2/1
  R1/1 -> Sum1/2
  Constant/1 -> Sum1/1
  Matrix Concatenate/1 -> Display/1, Math Function2/1  "J"
  Vector Concatenate1/1 -> Matrix Concatenate/2
  Vector Concatenate/1 -> Matrix Concatenate/1
  Trigonometric Function2/1 -> Gain/1, Vector Concatenate/2
  Gain/1 -> Vector Concatenate1/1
  Trigonometric Function2/2 -> Vector Concatenate/1, Vector Concatenate1/2
  Trigonometric Function1/1 -> Trigonometric Function2/1  "j"
  Selector3/1 -> Trigonometric Function1/2
  Selector2/1 -> Trigonometric Function1/1
  Trigonometric Function/1 -> Terminator/1  "alphas"
  Divide1/1 -> Trigonometric Function/1, R1/1  "lc"
  Selector1/1 -> Divide1/1
  Divide/1 -> Trigonometric Function/2, Switch/1, Switch/2, R2/1  "mu"
  R/1 -> Divide/2, Divide1/2
  w/1 -> Abs/1
  Arm/1 -> 3x3 Cross Product/2
  pqr/1 -> 3x3 Cross Product/1
  Sum of Elements/1 -> Sqrt/1
  Math Function/1 -> Sum of Elements/1
  Selector/1 -> Math Function/1
  Sum/1 -> Selector/1, Selector1/1, Selector2/1, Selector3/1  "Vr"
  Vb/1 -> Sum/2
  3x3 Cross Product/1 -> Sum/1

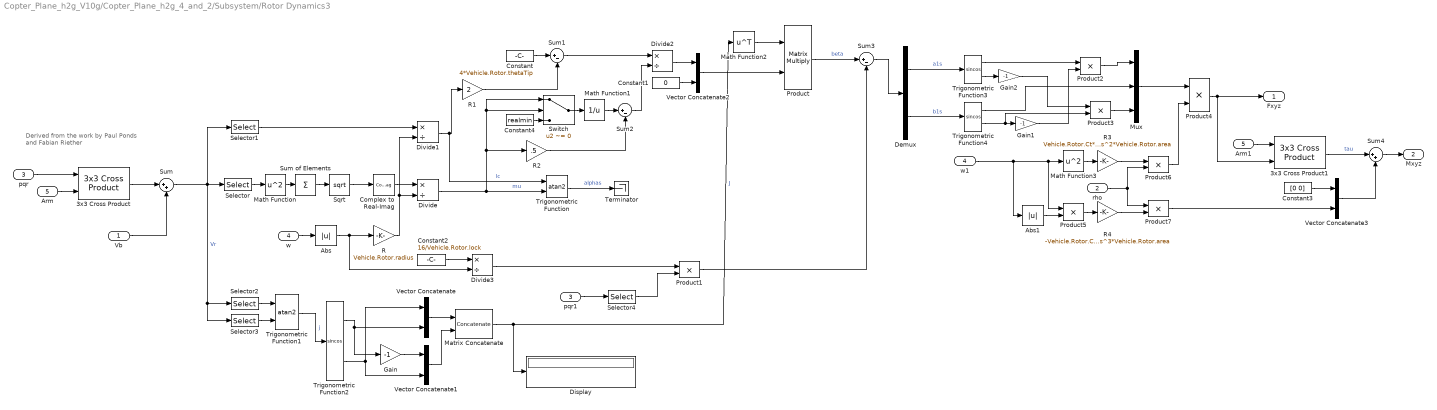
== system Copter_Plane_h2g_V10g/Copter_Plane_h2g_4_and_2/Subsystem/Rotor Dynamics3 ==
  note: Derived from the work by Paul Ponds
      | and Fabian Riether
  Vb : Inport  PortDimensions=3
  rho : Inport  Port=2  PortDimensions=1
  pqr : Inport  Port=3  PortDimensions=3
  w : Inport  Port=4  PortDimensions=[1 1]
  Arm : Inport  Port=5  PortDimensions=[3 1]
  3x3 Cross Product : sharedutil/3x3 Cross Product  aMode=aMode
      settings: SourceProductBaseCode=AE,PW,MT,UV,VE,VP
  3x3 Cross Product1 : sharedutil/3x3 Cross Product  aMode=aMode
      settings: SourceProductBaseCode=AE,PW,MT,UV,VE,VP
  Abs : Abs
  Abs1 : Abs
  Arm1 : InportShadow  Port=5  PortDimensions=[3 1]
  Complex to Real-Imag : ComplexToRealImag  Output=Real
  Constant : Constant  Value=4*Vehicle.Rotor.thetaTip
  Constant1 : Constant  Value=0
  Constant2 : Constant  Value=16/Vehicle.Rotor.lock
  Constant3 : Constant  Value=[0 0]
  Constant4 : Constant  Value=realmin
  Demux : Demux  Outputs=2
  Display : Display
  Divide{,1..3} (4 alike) : Product  Inputs=*/
  Gain : Gain  Gain=-1
  Gain1 : Gain  Gain=-1
  Gain2 : Gain  Gain=-1
  Math Function : Math  Operator=square  SignedPower=on  SaturateOnIntegerOverflow=on
  Math Function1 : Math  Operator=reciprocal  SignedPower=on  SaturateOnIntegerOverflow=on
  Math Function2 : Math  Operator=transpose  SignedPower=on  SaturateOnIntegerOverflow=on
  Math Function3 : Math  Operator=square  SignedPower=on  SaturateOnIntegerOverflow=on
  Matrix Concatenate : Concatenate  Mode=Multidimensional array  ConcatenateDimension=2
  Mux : Mux  Inputs=3
  Product : Product  Multiplication=Matrix(*)
  Product{1..7} (7 alike) : Product
  R : Gain  Gain=Vehicle.Rotor.radius
  R1 : Gain  Gain=2
  R2 : Gain  Gain=.5
  R3 : Gain  Gain=Vehicle.Rotor.Ct*Vehicle.Rotor.radius^2*Vehicle.Rotor.area
  R4 : Gain  Gain=-Vehicle.Rotor.Cq*Vehicle.Rotor.radius^3*Vehicle.Rotor.area
  Selector : Selector  InputPortWidth=3  IndexOptions=Index vector (dialog)  Indices=[1 2]  OutputSizes=1
  Selector1 : Selector  InputPortWidth=3  IndexOptions=Index vector (dialog)  Indices=[3]  OutputSizes=1
  Selector2 : Selector  InputPortWidth=3  IndexOptions=Index vector (dialog)  Indices=[2]  OutputSizes=1
  Selector3 : Selector  InputPortWidth=3  IndexOptions=Index vector (dialog)  Indices=[1]  OutputSizes=1
  Selector4 : Selector  InputPortWidth=3  IndexOptions=Index vector (dialog)  Indices=[2 1]  OutputSizes=1
  Sqrt : Sqrt  OutputSignalType=complex  SaturateOnIntegerOverflow=on
  Sum : Sum  Inputs=|++
  Sum of Elements : Sum  Inputs=+
  Sum1 : Sum  Inputs=|+-
  Sum2 : Sum  Inputs=|+-
  Sum3 : Sum  Inputs=|+-
  Sum4 : Sum  Inputs=|++
  Switch : Switch  Criteria=u2 ~= 0
  Terminator : Terminator
  Trigonometric Function : Trigonometry  Operator=atan2
  Trigonometric Function1 : Trigonometry  Operator=atan2
  Trigonometric Function2 : Trigonometry  Operator=sincos
  Trigonometric Function3 : Trigonometry  Operator=sincos
  Trigonometric Function4 : Trigonometry  Operator=sincos
  Vector Concatenate{,1..3} (4 alike) : Concatenate
  pqr1 : InportShadow  Port=3  PortDimensions=3
  w1 : InportShadow  Port=4  PortDimensions=[1 1]
  Fxyz : Outport  PortDimensions=[3 1]  VectorParamsAs1DForOutWhenUnconnected=off
  Mxyz : Outport  Port=2  PortDimensions=[3 1]  VectorParamsAs1DForOutWhenUnconnected=off
  wires:
  3x3 Cross Product/1 -> Sum/1
  Vb/1 -> Sum/2
  Sum/1 -> Selector3/1, Selector2/1, Selector1/1, Selector/1  "Vr"
  Selector/1 -> Math Function/1
  Math Function/1 -> Sum of Elements/1
  Sum of Elements/1 -> Sqrt/1
  pqr/1 -> 3x3 Cross Product/1
  Arm/1 -> 3x3 Cross Product/2
  w/1 -> Abs/1
  R/1 -> Divide1/2, Divide/2
  Divide/1 -> R2/1, Switch/2, Switch/1, Trigonometric Function/2  "mu"
  Selector1/1 -> Divide1/1
  Divide1/1 -> R1/1, Trigonometric Function/1  "lc"
  Trigonometric Function/1 -> Terminator/1  "alphas"
  Selector2/1 -> Trigonometric Function1/1
  Selector3/1 -> Trigonometric Function1/2
  Trigonometric Function1/1 -> Trigonometric Function2/1  "j"
  Trigonometric Function2/2 -> Vector Concatenate1/2, Vector Concatenate/1
  Gain/1 -> Vector Concatenate1/1
  Trigonometric Function2/1 -> Vector Concatenate/2, Gain/1
  Vector Concatenate/1 -> Matrix Concatenate/1
  Vector Concatenate1/1 -> Matrix Concatenate/2
  Matrix Concatenate/1 -> Math Function2/1, Display/1  "J"
  Constant/1 -> Sum1/1
  R1/1 -> Sum1/2
  Sum1/1 -> Divide2/1
  Math Function1/1 -> Sum2/1
  R2/1 -> Sum2/2
  Sum2/1 -> Divide2/2
  Divide2/1 -> Vector Concatenate2/1
  Constant1/1 -> Vector Concatenate2/2
  Vector Concatenate2/1 -> Product/2
  Math Function2/1 -> Product/1
  Product/1 -> Sum3/1  "beta"
  Constant2/1 -> Divide3/1
  pqr1/1 -> Selector4/1
  Selector4/1 -> Product1/2
  Abs/1 -> Divide3/2, R/1
  Divide3/1 -> Product1/1
  w1/1 -> Abs1/1, Product5/1, Math Function3/1
  Math Function3/1 -> R3/1
  Sum3/1 -> Demux/1
  Demux/1 -> Trigonometric Function3/1  "a1s"
  Demux/2 -> Trigonometric Function4/1  "b1s"
  Trigonometric Function4/2 -> Product3/2, Gain1/1
  Gain1/1 -> Product2/2
  Trigonometric Function3/1 -> Product2/1
  Product2/1 -> Mux/1
  Trigonometric Function4/1 -> Mux/2
  Trigonometric Function3/2 -> Gain2/1
  Product3/1 -> Mux/3
  Gain2/1 -> Product3/1
  Mux/1 -> Product4/1
  R3/1 -> Product6/1
  Abs1/1 -> Product5/2
  Product5/1 -> R4/1
  R4/1 -> Product7/2
  Constant3/1 -> Vector Concatenate3/1
  Vector Concatenate3/1 -> Sum4/2
  Arm1/1 -> 3x3 Cross Product1/1
  Product4/1 -> 3x3 Cross Product1/2, Fxyz/1
  3x3 Cross Product1/1 -> Sum4/1  "tau"
  Sum4/1 -> Mxyz/1
  Product6/1 -> Product4/2
  Product7/1 -> Vector Concatenate3/2
  rho/1 -> Product6/2, Product7/1
  Product1/1 -> Sum3/2
  Switch/1 -> Math Function1/1
  Constant4/1 -> Switch/3
  Sqrt/1 -> Complex to Real-Imag/1
  Complex to Real-Imag/1 -> Divide/1

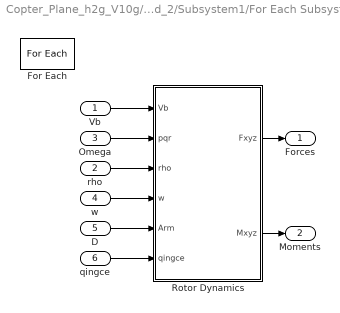
== system Copter_Plane_h2g_V10g/Copter_Plane_h2g_4_and_2/Subsystem1/For Each Subsystem ==
  Vb : Inport  PortDimensions=3
  rho : Inport  Port=2  PortDimensions=1
  Omega : Inport  Port=3
  w : Inport  Port=4  Partition=on  PartitionDimension=2  PartitionWidth=1  PartitionOffset=0
  D : Inport  Port=5  Partition=on  PartitionDimension=2  PartitionWidth=1  PartitionOffset=0
  qingce : Inport  Port=6  Partition=on  PartitionDimension=2  PartitionWidth=1  PartitionOffset=0
  For Each : ForEach  DisableCoverage=on
  Rotor Dynamics : Subsystem  AncestorBlock=dynamicsLibrary/Rotor Dynamics  TreatAsAtomicUnit=on
      mask init:
      | aeroicon('aeroblk');
      settings: RTWFcnNameOpts=Use subsystem name  RTWFileNameOpts=Use function name
  Forces : Outport  ConcatenationDimension=2  VectorParamsAs1DForOutWhenUnconnected=off
  Moments : Outport  Port=2  ConcatenationDimension=2  VectorParamsAs1DForOutWhenUnconnected=off
  wires:
  Rotor Dynamics/1(Fxyz) -> Forces/1
  Rotor Dynamics/2(Mxyz) -> Moments/1
  Vb/1 -> Rotor Dynamics/1(Vb)
  Omega/1 -> Rotor Dynamics/2(pqr)
  rho/1 -> Rotor Dynamics/3(rho)
  D/1 -> Rotor Dynamics/5(Arm)
  w/1 -> Rotor Dynamics/4(w)
  qingce/1 -> Rotor Dynamics/6(qingce)

== system Copter_Plane_h2g_V10g/Copter_Plane_h2g_4_and_2/Subsystem1/MotorsToW ==
  motors_datin : Inport
  Motordirections1 : Gain  Gain=[1 1 -1 -1]  ParamDataTypeStr=single  OutDataTypeStr=Inherit: Inherit via back propagation  SaturateOnIntegerOverflow=on
  Saturation5 : Saturate  UpperLimit=1  LowerLimit=realmin  OutDataTypeStr=Inherit: Inherit via back propagation
  motorsToW2_Gain : Gain  Gain=Vehicle.Motor.commandToWGain  ParamDataTypeStr=single  OutDataTypeStr=Inherit: Inherit via back propagation  SaturateOnIntegerOverflow=on
  motorsToW2_Gain1 : Gain  Gain=2*pi/60  ParamDataTypeStr=single  OutDataTypeStr=Inherit: Inherit via back propagation  SaturateOnIntegerOverflow=on
  omegas_datout : Outport  VectorParamsAs1DForOutWhenUnconnected=off
  wires:
  Saturation5/1 -> Motordirections1/1
  Motordirections1/1 -> motorsToW2_Gain/1
  motors_datin/1 -> Saturation5/1
  motorsToW2_Gain/1 -> motorsToW2_Gain1/1
  motorsToW2_Gain1/1 -> omegas_datout/1

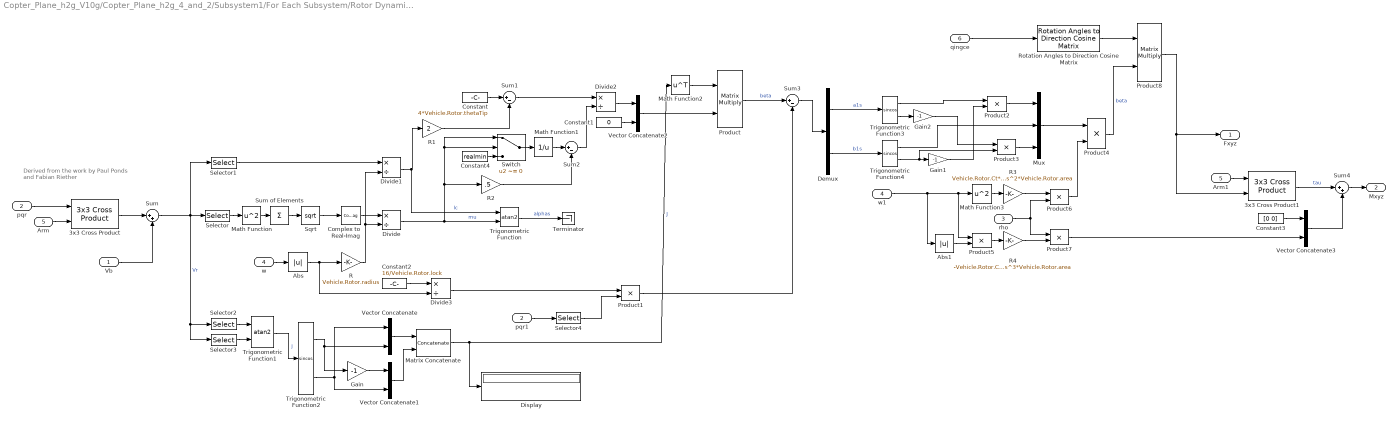
== system Copter_Plane_h2g_V10g/Copter_Plane_h2g_4_and_2/Subsystem1/For Each Subsystem/Rotor Dynamics ==
  note: Derived from the work by Paul Ponds
      | and Fabian Riether
  Vb : Inport  PortDimensions=3
  pqr : Inport  Port=2  PortDimensions=3
  rho : Inport  Port=3  PortDimensions=1
  w : Inport  Port=4  PortDimensions=[1 1]
  Arm : Inport  Port=5  PortDimensions=[3 1]
  qingce : Inport  Port=6  PortDimensions=[3 1]
  3x3 Cross Product : sharedutil/3x3 Cross Product  aMode=aMode
      settings: SourceProductBaseCode=AE,PW,MT,UV,VE,VP
  3x3 Cross Product1 : sharedutil/3x3 Cross Product  aMode=aMode
      settings: SourceProductBaseCode=AE,PW,MT,UV,VE,VP
  Abs : Abs
  Abs1 : Abs
  Arm1 : InportShadow  Port=5  PortDimensions=[3 1]
  Complex to Real-Imag : ComplexToRealImag  Output=Real
  Constant : Constant  Value=4*Vehicle.Rotor.thetaTip
  Constant1 : Constant  Value=0
  Constant2 : Constant  Value=16/Vehicle.Rotor.lock
  Constant3 : Constant  Value=[0 0]
  Constant4 : Constant  Value=realmin
  Demux : Demux  Outputs=2
  Display : Display
  Divide{,1..3} (4 alike) : Product  Inputs=*/
  Gain : Gain  Gain=-1
  Gain1 : Gain  Gain=-1
  Gain2 : Gain  Gain=-1
  Math Function : Math  Operator=square  SignedPower=on  SaturateOnIntegerOverflow=on
  Math Function1 : Math  Operator=reciprocal  SignedPower=on  SaturateOnIntegerOverflow=on
  Math Function2 : Math  Operator=transpose  SignedPower=on  SaturateOnIntegerOverflow=on
  Math Function3 : Math  Operator=square  SignedPower=on  SaturateOnIntegerOverflow=on
  Matrix Concatenate : Concatenate  Mode=Multidimensional array  ConcatenateDimension=2
  Mux : Mux  Inputs=3
  Product : Product  Multiplication=Matrix(*)
  Product{1..7} (7 alike) : Product
  Product8 : Product  Multiplication=Matrix(*)
  R : Gain  Gain=Vehicle.Rotor.radius
  R1 : Gain  Gain=2
  R2 : Gain  Gain=.5
  R3 : Gain  Gain=Vehicle.Rotor.Ct*Vehicle.Rotor.radius^2*Vehicle.Rotor.area
  R4 : Gain  Gain=-Vehicle.Rotor.Cq*Vehicle.Rotor.radius^3*Vehicle.Rotor.area
  Rotation Angles to Direction Cosine Matrix : sharedtransform/Rotation Angles to Direction Cosine Matrix  rotationOrder=YXZ  aMode=aMode
      settings: SourceProductBaseCode=AE,PW,MT,UV,VE,VP
  Selector : Selector  InputPortWidth=3  IndexOptions=Index vector (dialog)  Indices=[1 2]  OutputSizes=1
  Selector1 : Selector  InputPortWidth=3  IndexOptions=Index vector (dialog)  Indices=[3]  OutputSizes=1
  Selector2 : Selector  InputPortWidth=3  IndexOptions=Index vector (dialog)  Indices=[2]  OutputSizes=1
  Selector3 : Selector  InputPortWidth=3  IndexOptions=Index vector (dialog)  Indices=[1]  OutputSizes=1
  Selector4 : Selector  InputPortWidth=3  IndexOptions=Index vector (dialog)  Indices=[2 1]  OutputSizes=1
  Sqrt : Sqrt  OutputSignalType=complex  SaturateOnIntegerOverflow=on
  Sum : Sum  Inputs=|++
  Sum of Elements : Sum  Inputs=+
  Sum1 : Sum  Inputs=|+-
  Sum2 : Sum  Inputs=|+-
  Sum3 : Sum  Inputs=|+-
  Sum4 : Sum  Inputs=|++
  Switch : Switch  Criteria=u2 ~= 0
  Terminator : Terminator
  Trigonometric Function : Trigonometry  Operator=atan2
  Trigonometric Function1 : Trigonometry  Operator=atan2
  Trigonometric Function2 : Trigonometry  Operator=sincos
  Trigonometric Function3 : Trigonometry  Operator=sincos
  Trigonometric Function4 : Trigonometry  Operator=sincos
  Vector Concatenate{,1..3} (4 alike) : Concatenate
  pqr1 : InportShadow  Port=2  PortDimensions=3
  w1 : InportShadow  Port=4  PortDimensions=[1 1]
  Fxyz : Outport  PortDimensions=[3 1]  VectorParamsAs1DForOutWhenUnconnected=off
  Mxyz : Outport  Port=2  PortDimensions=[3 1]  VectorParamsAs1DForOutWhenUnconnected=off
  wires:
  Complex to Real-Imag/1 -> Divide/1
  Sqrt/1 -> Complex to Real-Imag/1
  Constant4/1 -> Switch/3
  Switch/1 -> Math Function1/1
  Product1/1 -> Sum3/2
  rho/1 -> Product7/1, Product6/2
  Product7/1 -> Vector Concatenate3/2
  Product6/1 -> Product4/2
  Sum4/1 -> Mxyz/1
  3x3 Cross Product1/1 -> Sum4/1  "tau"
  Arm1/1 -> 3x3 Cross Product1/1
  Vector Concatenate3/1 -> Sum4/2
  Constant3/1 -> Vector Concatenate3/1
  R4/1 -> Product7/2
  Product5/1 -> R4/1
  Abs1/1 -> Product5/2
  R3/1 -> Product6/1
  Mux/1 -> Product4/1
  Gain2/1 -> Product3/1
  Product3/1 -> Mux/3
  Trigonometric Function3/2 -> Gain2/1
  Trigonometric Function4/1 -> Mux/2
  Product2/1 -> Mux/1
  Trigonometric Function3/1 -> Product2/1
  Gain1/1 -> Product2/2
  Trigonometric Function4/2 -> Gain1/1, Product3/2
  Demux/2 -> Trigonometric Function4/1  "b1s"
  Demux/1 -> Trigonometric Function3/1  "a1s"
  Sum3/1 -> Demux/1
  Math Function3/1 -> R3/1
  w1/1 -> Math Function3/1, Product5/1, Abs1/1
  Divide3/1 -> Product1/1
  Abs/1 -> R/1, Divide3/2
  Selector4/1 -> Product1/2
  pqr1/1 -> Selector4/1
  Constant2/1 -> Divide3/1
  Product/1 -> Sum3/1  "beta"
  Math Function2/1 -> Product/1
  Vector Concatenate2/1 -> Product/2
  Constant1/1 -> Vector Concatenate2/2
  Divide2/1 -> Vector Concatenate2/1
  Sum2/1 -> Divide2/2
  R2/1 -> Sum2/2
  Math Function1/1 -> Sum2/1
  Sum1/1 -> Divide2/1
  R1/1 -> Sum1/2
  Constant/1 -> Sum1/1
  Matrix Concatenate/1 -> Display/1, Math Function2/1  "J"
  Vector Concatenate1/1 -> Matrix Concatenate/2
  Vector Concatenate/1 -> Matrix Concatenate/1
  Trigonometric Function2/1 -> Gain/1, Vector Concatenate/2
  Gain/1 -> Vector Concatenate1/1
  Trigonometric Function2/2 -> Vector Concatenate/1, Vector Concatenate1/2
  Trigonometric Function1/1 -> Trigonometric Function2/1  "j"
  Selector3/1 -> Trigonometric Function1/2
  Selector2/1 -> Trigonometric Function1/1
  Trigonometric Function/1 -> Terminator/1  "alphas"
  Divide1/1 -> Trigonometric Function/1, R1/1  "lc"
  Selector1/1 -> Divide1/1
  Divide/1 -> Trigonometric Function/2, Switch/1, Switch/2, R2/1  "mu"
  R/1 -> Divide/2, Divide1/2
  w/1 -> Abs/1
  Arm/1 -> 3x3 Cross Product/2
  pqr/1 -> 3x3 Cross Product/1
  Sum of Elements/1 -> Sqrt/1
  Math Function/1 -> Sum of Elements/1
  Selector/1 -> Math Function/1
  Sum/1 -> Selector/1, Selector1/1, Selector2/1, Selector3/1  "Vr"
  Vb/1 -> Sum/2
  3x3 Cross Product/1 -> Sum/1
  qingce/1 -> Rotation Angles to Direction Cosine Matrix/1
  Rotation Angles to Direction Cosine Matrix/1 -> Product8/1
  Product4/1 -> Product8/2  "beta"
  Product8/1 -> 3x3 Cross Product1/2, Fxyz/1

== matlab function Copter_Plane_h2g_V10g/Copter_Plane_h2g_4_and_2/MATLAB Function10 ==
  data: x_cmss input; forward output; y_cmss input; right output; yaw data_store_memory
function [forward, right]= to_body(  x_cmss,   y_cmss)  
global yaw
    forward = x_cmss * cos(yaw) + y_cmss * sin(yaw);
    right = -x_cmss * sin(yaw) + y_cmss * cos(yaw);

== matlab function Copter_Plane_h2g_V10g/Copter_Plane_h2g_4_and_2/MATLAB Function5 ==
  data: x_cmss input; forward output; y_cmss input; right output; yaw data_store_memory
function [forward, right]= to_body(  x_cmss,   y_cmss)  
global yaw
    forward = x_cmss * cos(yaw) + y_cmss * sin(yaw);
    right = -x_cmss * sin(yaw) + y_cmss * cos(yaw);

== matlab function Copter_Plane_h2g_V10g/Copter_Plane_h2g_4_and_2/MATLAB Function11 ==
  data: x_cmss input; forward output; y_cmss input; right output; yaw data_store_memory
function [forward, right]= to_body(  x_cmss,   y_cmss)  
global yaw
    forward = x_cmss * cos(yaw) + y_cmss * sin(yaw);
    right = -x_cmss * sin(yaw) + y_cmss * cos(yaw);

== matlab function Copter_Plane_h2g_V10g/Copter_Plane_h2g_4_and_2/MATLAB Function13 ==
  data: x_cmss input; forward output; y_cmss input; right output; yaw data_store_memory
function [forward, right]= to_body(  x_cmss,   y_cmss)  
global yaw
    forward = x_cmss * cos(yaw) + y_cmss * sin(yaw);
    right = -x_cmss * sin(yaw) + y_cmss * cos(yaw);

== matlab function Copter_Plane_h2g_V10g/Copter_Plane_h2g_4_and_2/MATLAB Function7 ==
  data: x_cmss input; forward output; y_cmss input; right output; yaw data_store_memory
function [forward, right]= to_body(  x_cmss,   y_cmss)  
global yaw
    forward = x_cmss * cos(yaw) + y_cmss * sin(yaw);
    right = -x_cmss * sin(yaw) + y_cmss * cos(yaw);

== matlab function Copter_Plane_h2g_V10g/Copter_Plane_h2g_4_and_2/MATLAB Function8 ==
  data: x_cmss input; forward output; y_cmss input; right output; yaw data_store_memory
function [forward, right]= to_body(  x_cmss,   y_cmss)  
global yaw
    forward = x_cmss * cos(yaw) + y_cmss * sin(yaw);
    right = -x_cmss * sin(yaw) + y_cmss * cos(yaw);

== matlab function Copter_Plane_h2g_V10g/Copter_Plane_h2g_4_and_2/MATLAB Function12 ==
  data: x_cmss input; forward output; y_cmss input; right output; yaw data_store_memory
function [forward, right]= to_body(  x_cmss,   y_cmss)  
global yaw
    forward = x_cmss * cos(yaw) + y_cmss * sin(yaw);
    right = -x_cmss * sin(yaw) + y_cmss * cos(yaw);
